simulink model "test_excitation_system_4a"  (R2025a)
settings: Solver=VariableStepAuto  StartTime=0.0  StopTime=10.0  RelTol=1e-3
libraries: spsExcitationSystemLib x1, spspowerguiLib x1
settings Model: Creator=adamsedlak  LastModifiedBy=adamsedlak

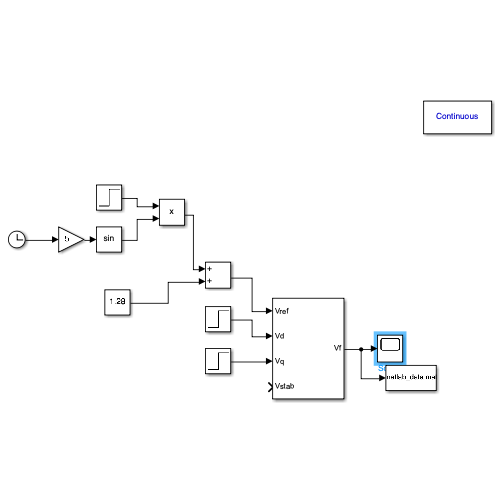
[thumbnail: Simulink's stored preview of the top-level diagram]
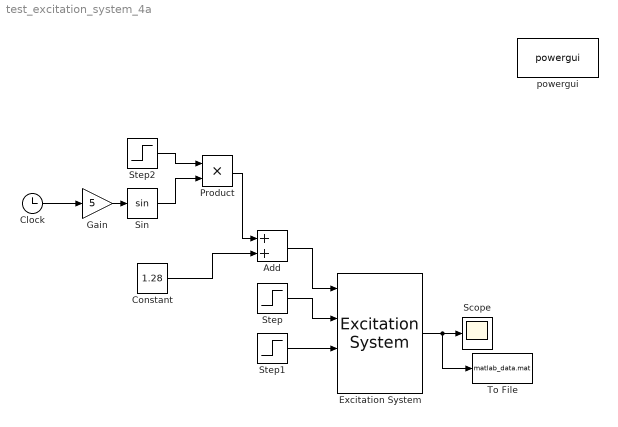
== system test_excitation_system_4a ==
  Add : Sum
  Clock : Clock
  Constant : Constant  Value=1.28
  Excitation System : spsExcitationSystemLib/Excitation System  tr=20e-3  reg=[ 300, 0.001 ]  exc=[ 1, 1.15]  tgr=[ 0.006, 0.173 ]  damp=[ 0.001, 0.1 ]  sat=[ 0, 0 ]  lim=[ -11.5, 11.5, 0 ]  v0=[1.28, 1.28]
      settings: LibrarySourceBlock=sps_lib/Electrical Machines/Synchronous Machine Control/Excitation System
  Gain : Gain  Gain=5
  Product : Product
  Scope : Scope
      settings: ActiveDisplayYMinimum=-5.7239605986413764  ActiveDisplayYMaximum=2.0583955350005958
  Sin : Trigonometry
  Step : Step  Before=1.28  After=1.3  SampleTime=0
  Step1 : Step  After=0.04  SampleTime=0
  Step2 : Step  After=0.001  SampleTime=0
  To File : ToFile  Filename=matlab_data.mat
  powergui : spspowerguiLib/powergui  Priority=1  SimulationMode=Continuous  SampleTime=50e-6  frequency=60  Iterations=50  frequencyindice=60  Pbase=100e6  ErrMax=1e-4  UnitsV=kV  UnitsW=MW  buscounter=0  FunctionMessages=off  echomessages=off  EnableUseOfTLC=off  CurrentSourceSwitches=off  DisableSnubberDevices=off  DisableRonSwitches=off  DisableVfSwitches=off  DisplayEquations=off  AutomaticDiscreteSolvers=off  SolverType=Tustin/Backward Euler (TBE)  Interpol=off  ExternalGateDelay=off  methode=off  Ts=100  x0status=blocks  SPID=on  SwTol=0  HookPort=off  NonlinearTolerance=1e-4  nMaxIteration=100  ContinueOnMaxIteration=off  RestoreLinks=warning  ResistiveCurrentMeasurement=off  Frange=[0:2:500]  Ylog=off  Xlog=on  ShowGrid=off  save=off  variable=ZData  structure=0  ZoomFFT=off  StartTime=0.0  cycles=1  DisplayStyle=1  fundamental=60  FreqAxis=off  MaxFrequency=1000  frequencyindicesteady=1  RmsSteady=1  display=off
  wires:
  Add/1 -> Excitation System/1
  Step/1 -> Excitation System/2
  Step1/1 -> Excitation System/3
  Excitation System/1 -> To File/1, Scope/1
  Constant/1 -> Add/2
  Clock/1 -> Gain/1
  Gain/1 -> Sin/1
  Sin/1 -> Product/2
  Step2/1 -> Product/1
  Product/1 -> Add/1
